simulink model "libdelta_conversion_simulink"  (R2023b)
settings: Solver=VariableStepAuto  StartTime=0.0  StopTime=10.0  RelTol=1e-3
settings Model: Creator=chris  LastModifiedBy=chris

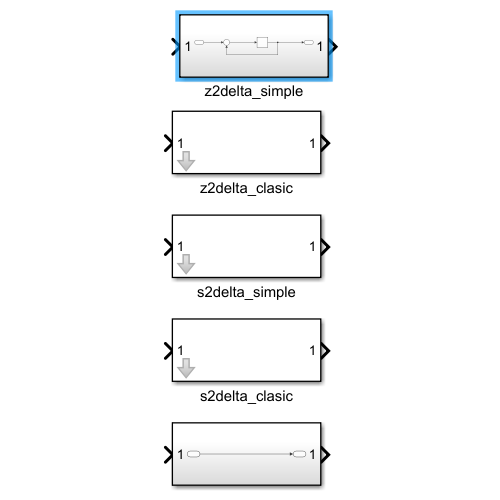
[thumbnail: Simulink's stored preview of the top-level diagram]
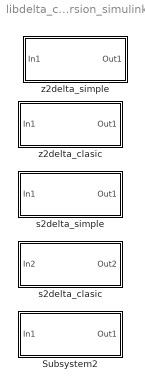
== system libdelta_conversion_simulink ==
  Subsystem2 : Subsystem
  s2delta_clasic : Subsystem  mask{T=0}
  s2delta_simple : Subsystem  mask{T=0}
  z2delta_clasic : Subsystem  mask{T=0}
  z2delta_simple : Subsystem

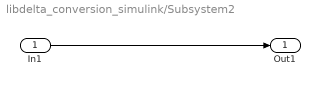
== system libdelta_conversion_simulink/Subsystem2 ==
  In1 : Inport
  Out1 : Outport
  wires:
  In1/1 -> Out1/1

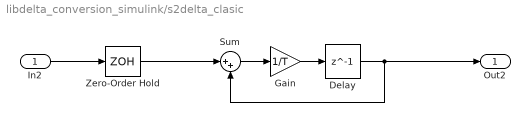
== system libdelta_conversion_simulink/s2delta_clasic ==
  In2 : Inport
  Delay : Delay  DelayLength=1  InitialCondition=0
  Gain : Gain  Gain=1/T
  Sum : Sum  Inputs=|++
  Zero-Order Hold : ZeroOrderHold  SampleTime=T
  Out2 : Outport
  wires:
  Zero-Order Hold/1 -> Sum/1
  In2/1 -> Zero-Order Hold/1
  Delay/1 -> Out2/1, Sum/2
  Sum/1 -> Gain/1
  Gain/1 -> Delay/1

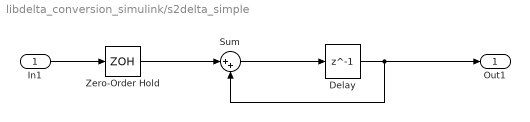
== system libdelta_conversion_simulink/s2delta_simple ==
  In1 : Inport
  Delay : Delay  DelayLength=1  InitialCondition=0
  Sum : Sum  Inputs=|++
  Zero-Order Hold : ZeroOrderHold  SampleTime=T
  Out1 : Outport
  wires:
  In1/1 -> Zero-Order Hold/1
  Sum/1 -> Delay/1
  Delay/1 -> Out1/1, Sum/2
  Zero-Order Hold/1 -> Sum/1

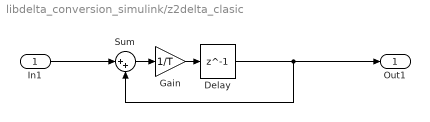
== system libdelta_conversion_simulink/z2delta_clasic ==
  In1 : Inport
  Delay : Delay  DelayLength=1  InitialCondition=0
  Gain : Gain  Gain=1/T
  Sum : Sum  Inputs=|++
  Out1 : Outport
  wires:
  In1/1 -> Sum/1
  Delay/1 -> Out1/1, Sum/2
  Sum/1 -> Gain/1
  Gain/1 -> Delay/1

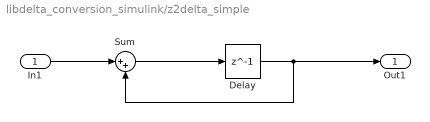
== system libdelta_conversion_simulink/z2delta_simple ==
  In1 : Inport
  Delay : Delay  DelayLength=1  InitialCondition=0
  Sum : Sum  Inputs=|++
  Out1 : Outport
  wires:
  In1/1 -> Sum/1
  Delay/1 -> Out1/1, Sum/2
  Sum/1 -> Delay/1
